simulink model "calc_B_FandMaero_th"  (R2020a)
settings: Solver=VariableStepAuto  StartTime=0.0  StopTime=0  RelTol=1e-3
values from neighbouring files (symbols this model uses):
  rollVal = 5*pi/180    (= 0.0872664625997)    [calc_B_FandMaero_ts.m]
  testAoA = 5    [calc_B_FandMaero_ts.m]
  vApp = [-10;0;0]    [calc_B_FandMaero_ts.m]
libraries: calc_B_FandMaero x1
settings Model: Creator=Ayaz  LastModifiedBy=Ayaz

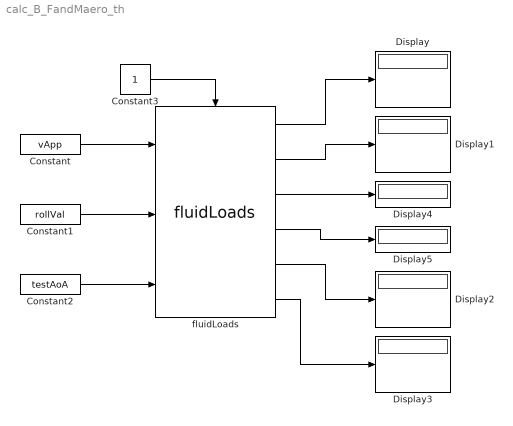
== system calc_B_FandMaero_th ==
  Constant : Constant  Value=vApp  VectorParams1D=off
  Constant1 : Constant  Value=rollVal  VectorParams1D=off
  Constant2 : Constant  Value=testAoA  VectorParams1D=off
  Constant3 : Constant
  Display{,1..5} (6 alike) : Display
  fluidLoads : calc_B_FandMaero/fluidLoads  refArea=Sref  aeroCent=[-1;0;0]  flowDensity=rho  AoA_vals=AoA_vals  CL_vals=CL_vals  CD_vals=CD_vals
  wires:
  Constant/1 -> fluidLoads/1
  Constant1/1 -> fluidLoads/2
  Constant2/1 -> fluidLoads/3
  fluidLoads/1 -> Display/1
  fluidLoads/2 -> Display1/1
  fluidLoads/5 -> Display2/1
  fluidLoads/6 -> Display3/1
  fluidLoads/4 -> Display5/1
  fluidLoads/3 -> Display4/1
  Constant3/1 -> fluidLoads/Enable
